simulink model "NLSys"  (R2018b)
settings: Solver=VariableStepAuto  StartTime=0.0  StopTime=10.0  RelTol=1e-3
PreLoadFcn:
  | lam = 1;
  | PL = 1;
  | gammaX = 1;
  | gammaR = 1;
  | Am = 0.8;
  | tau = 1;
  | K0x = (-1/tau - Am)/lam;
  | K0r = (1/tau)/lam;
  | 
  | Nu = 2;
  | T0 = 0;
  | Tf = 10;
  | time = [T0;Tf];
  | Nt = length(time);
  | data = zeros(Nt,Nu);
  | simin = [time data];
settings Model: Creator=Jyot Buch  LastModifiedBy=Jyot Buch

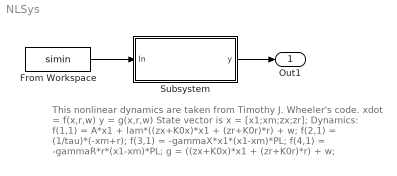
== system NLSys ==
  note: This nonlinear dynamics are taken from Timothy J. Wheeler's code.
      | xdot = f(x,r,w)
      | y = g(x,r,w)
      |
      | State vector is
      | x = [x1;xm;zx;zr];
      |
      | Dynamics:
      | f(1,1) = A*x1 + lam*((zx+K0x)*x1 + (zr+K0r)*r) + w;
      | f(2,1) = (1/tau)*(-xm+r);
      | f(3,1) = -gammaX*x1*(x1-xm)*PL;
      | f(4,1) = -gammaR*r*(x1-xm)*PL;
      | g = ((zx+K0x)*x1 + (zr+K0r)*r) + w;
  From Workspace : FromWorkspace  VariableName=simin  SampleTime=0
  Subsystem : Subsystem
  Out1 : Outport
  wires:
  From Workspace/1 -> Subsystem/1(In)
  Subsystem/1(y) -> Out1/1

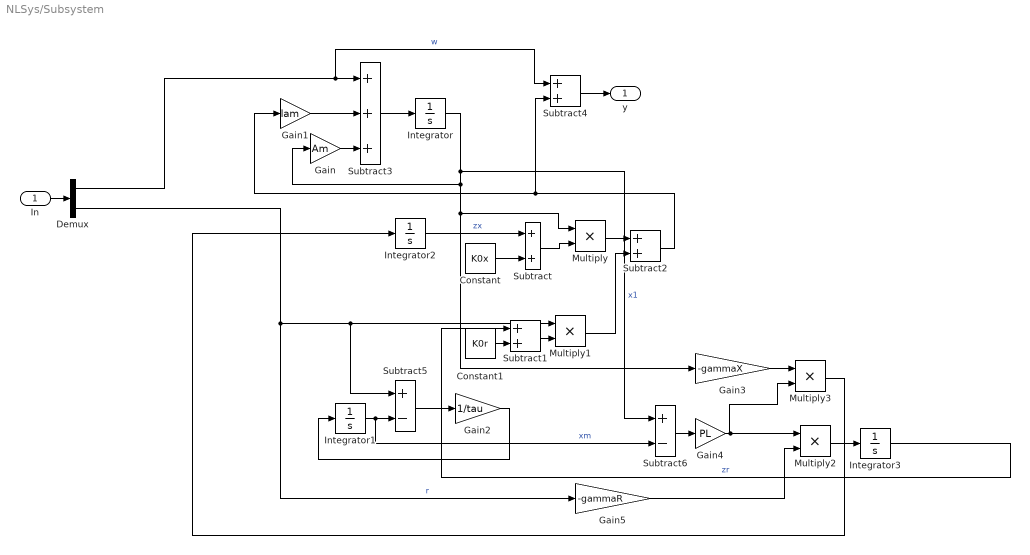
== system NLSys/Subsystem ==
  In : Inport
  Constant : Constant  Value=K0x
  Constant1 : Constant  Value=K0r
  Demux : Demux  Outputs=2
  Gain : Gain  Gain=Am
  Gain1 : Gain  Gain=lam
  Gain2 : Gain  Gain=1/tau
  Gain3 : Gain  Gain=-gammaX
  Gain4 : Gain  Gain=PL
  Gain5 : Gain  Gain=-gammaR
  Integrator{,1..3} (4 alike) : Integrator
  Multiply{,1..3} (4 alike) : Product
  Subtract{,1..2,4} (4 alike) : Sum
  Subtract3 : Sum  Inputs=+++
  Subtract5 : Sum  Inputs=+-
  Subtract6 : Sum  Inputs=+-
  y : Outport
  wires:
  Integrator/1 -> Gain3/1, Multiply/1, Gain/1, Subtract6/1  "x1"
  Integrator1/1 -> Subtract6/2, Subtract5/2  "xm"
  Integrator2/1 -> Subtract/1  "zx"
  Integrator3/1 -> Subtract1/1  "zr"
  Multiply3/1 -> Integrator2/1
  Constant/1 -> Subtract/2
  Subtract/1 -> Multiply/2
  Constant1/1 -> Subtract1/2
  Subtract1/1 -> Multiply1/2
  Demux/2 -> Gain5/1, Subtract5/1, Multiply1/1  "r"
  Multiply/1 -> Subtract2/1
  Multiply1/1 -> Subtract2/2
  Subtract2/1 -> Subtract4/2, Gain1/1
  Subtract3/1 -> Integrator/1
  Demux/1 -> Subtract4/1, Subtract3/1  "w"
  Gain1/1 -> Subtract3/2
  Gain/1 -> Subtract3/3
  Subtract4/1 -> y/1
  Subtract5/1 -> Gain2/1
  Gain2/1 -> Integrator1/1
  Subtract6/1 -> Gain4/1
  Gain4/1 -> Multiply3/2, Multiply2/1
  Gain5/1 -> Multiply2/2
  Gain3/1 -> Multiply3/1
  Multiply2/1 -> Integrator3/1
  In/1 -> Demux/1
